simulink model "FOC_PMSM"  (R2024b)
settings: Solver=ode5  StartTime=0.0  StopTime=T  FixedStep=Tsim  RelTol=1e-3
InitFcn:
  | T = 0.6;
  | Tsim = 1e-6;
  | Tcarrier = 50e-6; % fcarrier = 20kHz
  | 
  | % Treal is used to simulate
  | % real-world conditions of the MCU
  | %------------------------------
  | Treal = 25e-6;
  | 
  | % 2*Tspeed is set for the speed-loop
  | % PI controller and is slower than
  | % the current-loop PI controller
  | %--------------------------------
  | 
  | %Init:
  | % Rs = 0.62 (Ohm)
  | % Ls = 0.002075 (H)
  | % J = 36.17e-05 (kg*m^2)
  | % B = 9.444e-05 (N.m.s)
  | % K_t = 1.5*np*psi_m
  | %     = 0.51762 (N*m/A)
  |     %psi_m: flux leakage
  | % Rated currernt:
  | %   Iq = Te/Kt = 11.59A
  | 
  | np = 4;
  | ff_gain = 1;
  | 
  | %Current Loop:
  | Kp_current = 80 ;
  | Ki_current = 100 ;
  | 
  | %Speed Loop:
  | Kp_speed = 0.5;
  | Ki_speed = 30;
  | 
  | %Position Loop:
  | Kp_position = 100;
  | 
  | %====== Adaptive Fuzzy PI ========
  | um = 1;
  | em = 12;
  | D_em = 1.8;
  | 
  | kappa = 0.8;
  | epsilon = 0.01;
  | 
  | alpha = 20;
  | beta = 25;
undefined symbols (not defined in the file or in its folder): DiscIntNeverNeededParam
libraries: spsMosfetLib x12, slpidlib x8, eeTransforms x4, simulink x4, spsDCVoltageSourceLib x2, spsPermanentMagnetSynchronousMachineLib x2, SignalEditorBlockLib x2, fuzblock x1, sps_lib x1
(part 2 of 2)

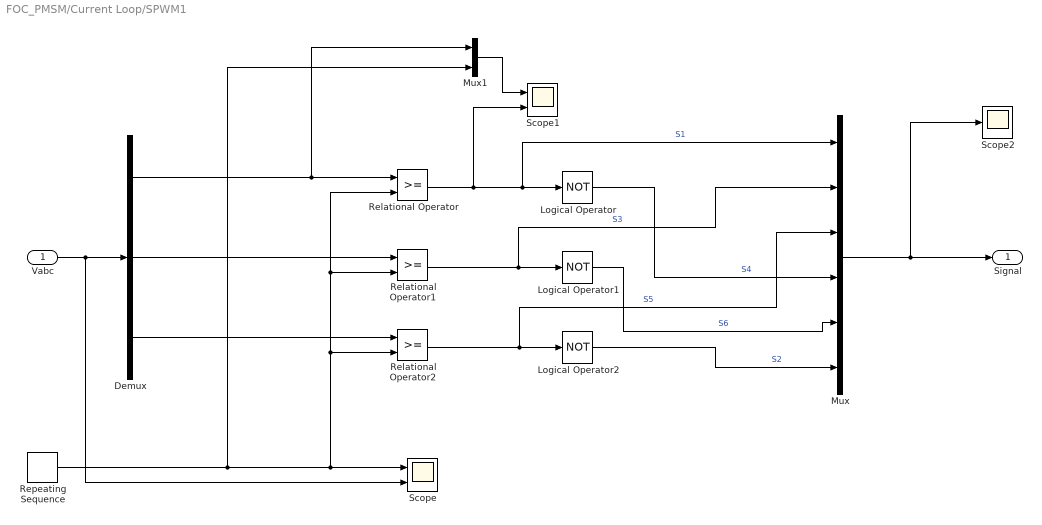
== system FOC_PMSM/Current Loop/SPWM1 ==
  Vabc : Inport
  Demux : Demux  Outputs=3
  Logical Operator : Logic  Operator=NOT  AllPortsSameDT=off  OutDataTypeStr=boolean
  Logical Operator1 : Logic  Operator=NOT  AllPortsSameDT=off  OutDataTypeStr=boolean
  Logical Operator2 : Logic  Operator=NOT  AllPortsSameDT=off  OutDataTypeStr=boolean
  Mux : Mux  Inputs=6
  Mux1 : Mux  Inputs=2
  Relational Operator : RelationalOperator  OutDataTypeStr=boolean  RndMeth=Simplest  InputSameDT=off
  Relational Operator1 : RelationalOperator  OutDataTypeStr=boolean  RndMeth=Simplest  InputSameDT=off
  Relational Operator2 : RelationalOperator  OutDataTypeStr=boolean  RndMeth=Simplest  InputSameDT=off
  Repeating Sequence : simulink/Sources/Repeating Sequence  rep_seq_t=[0, 0.5*Tcarrier, Tcarrier]  rep_seq_y=[-150, 150, -150]
  Scope : Scope  NumInputPorts=2
  Scope1 : Scope  NumInputPorts=2
  Scope2 : Scope
  Signal : Outport
  wires:
  Mux1/1 -> Scope1/1
  Mux/1 -> Signal/1, Scope2/1
  Logical Operator2/1 -> Mux/6  "S2"
  Logical Operator1/1 -> Mux/5  "S6"
  Logical Operator/1 -> Mux/4  "S4"
  Relational Operator2/1 -> Logical Operator2/1, Mux/3  "S5"
  Relational Operator1/1 -> Logical Operator1/1, Mux/2  "S3"
  Relational Operator/1 -> Logical Operator/1, Mux/1, Scope1/2  "S1"
  Demux/3 -> Relational Operator2/1
  Demux/2 -> Relational Operator1/1
  Repeating Sequence/1 -> Scope/1, Relational Operator2/2, Relational Operator1/2, Relational Operator/2, Mux1/2
  Demux/1 -> Relational Operator/1, Mux1/1
  Vabc/1 -> Demux/1, Scope/2

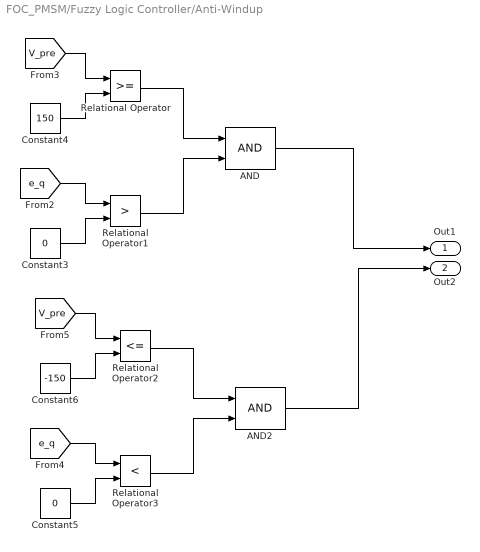
== system FOC_PMSM/Fuzzy Logic Controller/Anti-Windup ==
  AND : Logic  IconShape=distinctive  AllPortsSameDT=off  OutDataTypeStr=boolean
  AND2 : Logic  IconShape=distinctive  AllPortsSameDT=off  OutDataTypeStr=boolean
  Constant3 : Constant  Value=0
  Constant4 : Constant  Value=150
  Constant5 : Constant  Value=0
  Constant6 : Constant  Value=-150
  Relational Operator : RelationalOperator  OutDataTypeStr=boolean  RndMeth=Simplest  InputSameDT=off
  Relational Operator1 : RelationalOperator  Operator=>  OutDataTypeStr=boolean  RndMeth=Simplest  InputSameDT=off
  Relational Operator2 : RelationalOperator  Operator=<=  OutDataTypeStr=boolean  RndMeth=Simplest  InputSameDT=off
  Relational Operator3 : RelationalOperator  Operator=<  OutDataTypeStr=boolean  RndMeth=Simplest  InputSameDT=off
  Out1 : Outport
  Out2 : Outport  Port=2
  wires:
  Relational Operator3/1 -> AND2/2
  [e_q] -> Relational Operator1/1
  Constant6/1 -> Relational Operator2/2
  [V_pre] -> Relational Operator2/1
  Constant3/1 -> Relational Operator1/2
  Constant4/1 -> Relational Operator/2
  Relational Operator2/1 -> AND2/1
  AND2/1 -> Out2/1
  [V_pre] -> Relational Operator/1
  Constant5/1 -> Relational Operator3/2
  Relational Operator/1 -> AND/1
  [e_q] -> Relational Operator3/1
  AND/1 -> Out1/1
  Relational Operator1/1 -> AND/2

== matlab function FOC_PMSM/Fuzzy Logic Controller/contraction-expansion  ==
  data: mu1 input; E_tilde output; mu2 input; kappa input; epsilon input; dE_tilde output
function [E_tilde, dE_tilde] = fcn(mu1, mu2, kappa, epsilon)
    % [Suy luận]: Tính hệ số co giãn lambda cho từng nhánh
    % mu_m mặc định bằng 1 trong hệ chuẩn hóa
    
    lambda1 = (abs(mu1))^kappa + epsilon;
    lambda2 = (abs(mu2))^kappa + epsilon;
    
    % [Suy luận]: Phóng đại tín hiệu đầu vào cho khối Fuzzy
    E_tilde = mu1 / lambda1;
    dE_tilde = mu2 / lambda2;
end
